simulink model "SimulinkPID"  (Simulink 8.7)
settings: Solver=FixedStepAuto  SolverMode=SingleTasking  StartTime=0.0  StopTime=0.005  RelTol=1e-3
libraries: simulink x1
settings Model: Creator=tmax4  LastModifiedBy=tmax4
settings DataIOCC: LimitDataPoints=off  SaveFormat=Dataset
settings OptimizationCC: DefaultParameterBehavior=Inlined  UseDivisionForNetSlopeComputation=on  UseFloatMulNetSlope=on  InlineInvariantSignals=on  PassReuseOutputArgsAs=Individual arguments  ZeroExternalMemoryAtStartup=off  ZeroInternalMemoryAtStartup=off  NoFixptDivByZeroProtection=on  EfficientFloat2IntCast=on  OptimizeModelRefInitCode=on  LifeSpan=1
settings DebuggingCC: UnderspecifiedInitializationDetection=Simplified  MergeDetectMultiDrivingBlocksExec=error
settings HardwareCC: ProdBitPerInt=16  ProdBitPerPointer=16  ProdIntDivRoundTo=Zero  ProdEndianess=LittleEndian  ProdWordSize=16  ProdHWDeviceType=Microchip->dsPIC
settings ModelReferenceCC: PropagateSignalLabelsOutOfModel=on
settings RTWCC: SystemTargetFile=ert.tlc  TemplateMakefile=ert_default_tmf  Description=Embedded Coder  GenerateReport=on  IncludeHyperlinkInReport=on  LaunchReport=on  GenerateTraceInfo=on  GenerateTraceReport=on  GenerateTraceReportSl=on  GenerateTraceReportSf=on  GenerateTraceReportEml=on  GenerateCodeMetricsReport=on
settings CodeAppCC: ForceParamTrailComments=on  IgnoreCustomStorageClasses=off  OperatorAnnotations=on  SimulinkDataObjDesc=on  SFDataObjDesc=on  MATLABFcnDesc=on  CustomSymbolStrGlobalVar=rt$N$M  CustomSymbolStrType=$N$M  CustomSymbolStrFcn=$N$M$F  CustomSymbolStrMacro=$N$M  InsertBlockDesc=on  MATLABSourceComments=on
settings ERTTargetCC: MultiwordLength=2048  GenerateSampleERTMain=on  IncludeMdlTerminateFcn=off  CombineSignalStateStructs=on  SupportComplex=off  SupportContinuousTime=on  InlinedParameterPlacement=NonHierarchical  ERTCustomFileTemplate=example_file_process.tlc  ERTFilePackagingFormat=CompactWithDataFile
settings ConfigComp: CovModelRefEnable=off

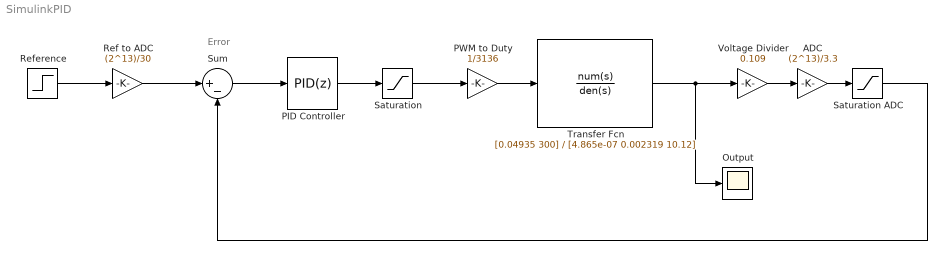
== system SimulinkPID ==
  note: Error
  ADC : Gain  Gain=(2^13)/3.3  OutDataTypeStr=uint16
  Output : Scope
  PID Controller : simulink/Continuous/PID Controller  Controller=PID  TimeDomain=Discrete-time  SampleTime=6.66e-6  IntegratorMethod=Trapezoidal  FilterMethod=Forward Euler  Form=Parallel  UseFilter=off  ControllerParametersSource=internal  P=5  I=40000  D=0.000006  N=0.009092182911359  InitialConditionSource=internal  InitialConditionForIntegrator=0  InitialConditionForFilter=0  ExternalReset=none  LimitOutput=off  UpperSaturationLimit=inf  LowerSaturationLimit=-inf  LinearizeAsGain=on  AntiWindupMode=none  Kb=1  TrackingMode=off  Kt=1  PParamMin=[]  PParamMax=[]  PParamDataTypeStr=int16  IParamMin=[]  IParamMax=[]  IParamDataTypeStr=int32  DParamMin=[]  DParamMax=[]  DParamDataTypeStr=int16  NParamMin=[]  NParamMax=[]  KbParamMin=[]  KbParamMax=[]  KtParamMin=[]  KtParamMax=[]  POutMin=[]  POutMax=[]  POutDataTypeStr=int32  PGainOutDataTypeStr=int32  PProdOutDataTypeStr=int32  IOutMin=[]  IOutMax=[]  IOutDataTypeStr=int32  IGainOutDataTypeStr=int32  IProdOutDataTypeStr=int32  DOutMin=[]  DOutMax=[]  DOutDataTypeStr=int32  DGainOutDataTypeStr=int32  DProdOutDataTypeStr=int32  NOutMin=[]  NOutMax=[]  KbOutMin=[]  KbOutMax=[]  KtOutMin=[]  KtOutMax=[]  IntegratorOutMin=[]  IntegratorOutMax=[]  IntegratorOutDataTypeStr=int32  FilterOutMin=[]  FilterOutMax=[]  SumOutMin=[]  SumOutMax=[]  SumOutDataTypeStr=int32  SumI1OutMin=[]  SumI1OutMax=[]  SumI2OutMin=[]  SumI2OutMax=[]  SumI3OutMin=[]  SumI3OutMax=[]  SumDOutMin=[]  SumDOutMax=[]  SumAccumDataTypeStr=int32  SaturationOutMin=[]  SaturationOutMax=[]  IntegratorContinuousStateAttributes=''  IntegratorStateMustResolveToSignalObject=off  IntegratorRTWStateStorageClass=Auto  FilterContinuousStateAttributes=''  FilterStateMustResolveToSignalObject=off  FilterRTWStateStorageClass=Auto  DifferentiatorICPrevScaledInput=0  DifferentiatorOutMin=[]  DifferentiatorOutMax=[]  DifferentiatorOutDataTypeStr=int32
  PWM to Duty : Gain  Gain=1/3136  OutDataTypeStr=double
  Ref to ADC : Gain  Gain=(2^13)/30  OutDataTypeStr=uint16
  Reference : Step  Time=0  After=10  SampleTime=0
  Saturation : Saturate  UpperLimit=2822  LowerLimit=62  OutDataTypeStr=uint16
  Saturation ADC : Saturate  UpperLimit=2^13  LowerLimit=0  OutDataTypeStr=uint16
  Sum : Sum  Inputs=|+-  OutDataTypeStr=int16
  Transfer Fcn : TransferFcn  Numerator=[0.04935 300]  Denominator=[4.865e-07 0.002319 10.12]
  Voltage Divider : Gain  Gain=0.109  OutDataTypeStr=double
  wires:
  Reference/1 -> Ref to ADC/1
  Sum/1 -> PID Controller/1
  Ref to ADC/1 -> Sum/1
  Saturation ADC/1 -> Sum/2
  PID Controller/1 -> Saturation/1
  Saturation/1 -> PWM to Duty/1
  Voltage Divider/1 -> ADC/1
  ADC/1 -> Saturation ADC/1
  Transfer Fcn/1 -> Output/1, Voltage Divider/1
  PWM to Duty/1 -> Transfer Fcn/1
